simulink model "sf_power_window"  (R2017b)
settings: Solver=FixedStepDiscrete  StartTime=0.0  StopTime=inf  FixedStep=0.1  RelTol=1e-3  EnableMultiTasking=on
PreLoadFcn:
  | %addpath([matlabroot '/toolbox/stateflow/sfdemos']);
  | %addpath([matlabroot '/toolbox/dsp/dsp']);
  | load sf_power_window_buses;
libraries: dspquant2 x1
settings Model: Creator=The MathWorks, Inc.  LastModifiedBy=The MathWorks, Inc.
settings DataIOCC: LimitDataPoints=on  SaveFormat=Array
settings OptimizationCC: LifeSpan=inf
settings DebuggingCC: SolverPrmCheckMsg=warning  AllowSymbolicDim=off  SFUnexpectedBacktrackingDiag=warning  SFNoUnconditionalDefaultTransitionDiag=warning  SFExecutionAtInitializationDiag=none
settings HardwareCC: ProdBitPerPointer=32  ProdBitPerSizeT=32  ProdBitPerPtrDiffT=32  ProdLargestAtomicFloat=None  ProdIntDivRoundTo=Undefined  ProdEndianess=Unspecified  ProdWordSize=32  ProdHWDeviceType=32-bit Generic
settings ModelReferenceCC: PropagateSignalLabelsOutOfModel=off
settings CodeAppCC: StateflowObjectComments=on
settings GRTTargetCC: TargetLangStandard=C89/C90 (ANSI)  GeneratePreprocessorConditionals=Disable all
settings ConfigComp: CovMetricSettings=dw  CovHtmlReporting=on  CovSaveCumulativeToWorkspaceVar=on  CovSaveSingleToWorkspaceVar=on  CovExternalEMLEnable=off  CovSFcnEnable=off

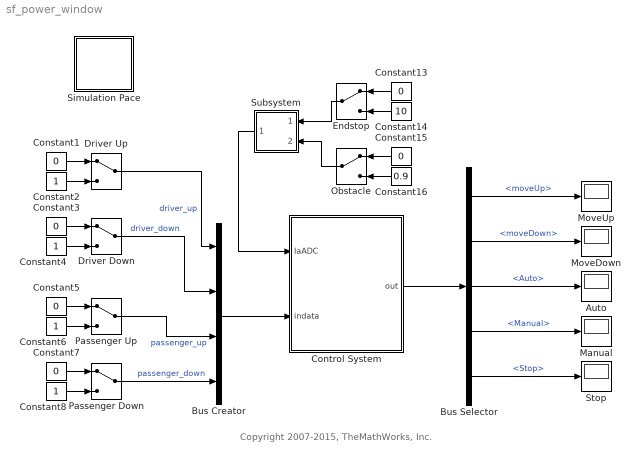
== system sf_power_window ==
  note: Copyright 2007-2015, TheMathWorks, Inc.
  Auto : Display
  Bus Creator : BusCreator  Inputs=4  OutDataTypeStr=Bus: in_busobj  NonVirtualBus=on
  Bus Selector : BusSelector  DialogController=Simulink.DDGSource_BusSelector  OutputSignals=moveUp,moveDown,Auto,Manual,Stop
  Constant{1,3,5,7} (4 alike) : Constant  Value=0  OutDataTypeStr=boolean
  Constant13 : Constant  Value=0
  Constant14 : Constant  Value=10
  Constant15 : Constant  Value=0
  Constant16 : Constant  Value=0.9
  Constant{2,4,6,8} (4 alike) : Constant  OutDataTypeStr=boolean
  Control System : Stateflow chart  TreatAsAtomicUnit=on
  Driver Down : ManualSwitch
  Driver Up : ManualSwitch
  Endstop : ManualSwitch
  Manual : Display
  MoveDown : Display
  MoveUp : Display
  Obstacle : ManualSwitch
  Passenger Down : ManualSwitch
  Passenger Up : ManualSwitch
  Simulation Pace : MATLAB Function  TreatAsAtomicUnit=on
  Stop : Display
  Subsystem : Subsystem
  wires:
  Constant13/1 -> Endstop/1
  Constant14/1 -> Endstop/2
  Constant15/1 -> Obstacle/1
  Constant16/1 -> Obstacle/2
  Endstop/1 -> Subsystem/1(In1)
  Obstacle/1 -> Subsystem/2(In2)
  Constant1/1 -> Driver Up/1
  Constant2/1 -> Driver Up/2
  Constant3/1 -> Driver Down/1
  Constant4/1 -> Driver Down/2
  Constant5/1 -> Passenger Up/1
  Constant6/1 -> Passenger Up/2
  Constant7/1 -> Passenger Down/1
  Constant8/1 -> Passenger Down/2
  Driver Up/1 -> Bus Creator/1  "driver_up"
  Driver Down/1 -> Bus Creator/2  "driver_down"
  Passenger Up/1 -> Bus Creator/3  "passenger_up"
  Passenger Down/1 -> Bus Creator/4  "passenger_down"
  Bus Creator/1 -> Control System/2(indata)
  Subsystem/1(Out1) -> Control System/1(IaADC)
  Control System/1(out) -> Bus Selector/1
  Bus Selector/1 -> MoveUp/1  "<moveUp>"
  Bus Selector/2 -> MoveDown/1  "<moveDown>"
  Bus Selector/3 -> Auto/1  "<Auto>"
  Bus Selector/4 -> Manual/1  "<Manual>"
  Bus Selector/5 -> Stop/1  "<Stop>"

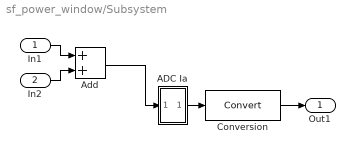
== system sf_power_window/Subsystem ==
  In1 : Inport
  In2 : Inport  Port=2
  ADC Ia : Subsystem  mask(AD Converter){Ts=0.01, peak=3.5, Td=0.005, bits=8}
      mask prompts: Ts "sample time (-1 for inherited)"; Td "delay (-1 for inherited)"
      mask help: Analog (A) to digital (D) converter with sample rate, conversion delay, range, and number of bits used for conversion.
      mask Display:
      | plot([0.5 1.5 1.5 2.5 2.5 3.5 3.5 4.5], [0 0 1 1 2 2 3 3])
      | plot([0 3], [0 3])
  Add : Sum
  Conversion : DataTypeConversion  ConvertRealWorld=Stored Integer (SI)  RndMeth=Nearest  SaturateOnIntegerOverflow=on
  Out1 : Outport
  wires:
  Add/1 -> ADC Ia/1(A)
  ADC Ia/1(D) -> Conversion/1
  In1/1 -> Add/1
  In2/1 -> Add/2
  Conversion/1 -> Out1/1

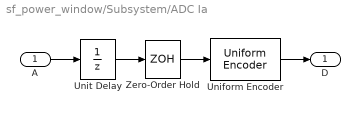
== system sf_power_window/Subsystem/ADC Ia ==
  A : Inport
  Uniform Encoder : dspquant2/Uniform Encoder  peak=peak  bits=bits  otype=Signed integer
      settings: SourceProductName=DSP System Toolbox
  Unit Delay : UnitDelay  SampleTime=0.1
  Zero-Order Hold : ZeroOrderHold  SampleTime=0.1
  D : Outport
  wires:
  A/1 -> Unit Delay/1
  Unit Delay/1 -> Zero-Order Hold/1
  Zero-Order Hold/1 -> Uniform Encoder/1
  Uniform Encoder/1 -> D/1

== matlab function sf_power_window/Simulation Pace ==
function fcn()
pause(0.1);

== stateflow chart sf_power_window/Control System ==
  state Switch [parallel]
    du: switches();
    settings: executionOrder=1
  state Logic [parallel]
    settings: executionOrder=2
    note: Remain in Stop state until a NEUTRAL event triggers Stop.Mode to be Ready.
        | Fail safe time out after continuous movement of more than five seconds.
    state Stop
      en:go.neutral();
      en:out.Stop=true;
      ex:out.Stop=false;
      state Mode [parallel]
        settings: executionOrder=1
        state Waiting
        state Ready
        (default) -> Waiting
        Waiting -> Ready : NEUTRAL
      state Position [parallel]
        settings: executionOrder=2
        state NotSureWhere
        state NearTop
        state NearBottom
        (default) -> NotSureWhere
        (junction 38) -> NearTop [order 1] : [in(EndStop.AtTop)]
        (junction 38) -> NearBottom [order 2]
    state go [group]
      state up [function]
        (default) -> (junction 123) : {out.moveDown = false;
            |  out.moveUp = true;}
      state neutral [function]
        (default) -> (junction 129) : {out.moveUp = false;
            |  out.moveDown = false;}
      state down [function]
        (default) -> (junction 126) : {out.moveUp = false;
            |  out.moveDown = true;}
    state EmergencyDown
      en: go.down();
    state Move
      en: obstacles.init();
      du: obstacles.detect();
      state obstacles [group]
        state detect [function]
          (default) -> (junction 134) : { newIa = cast(Ia*fi(0.96875,1,16,8) + IaADC*fi(0.03125,1,16,8), 'like', newIa);
              |   dIa = newIa-Ia;
              |   Ia = newIa;}
          (junction 134) -> (junction 135) [order 1] : [out.moveUp && Ia > 0.9]
          (junction 135) -> (junction 140) [order 1] : [(dIa >= 0.1)]  % top endstop
          (junction 134) -> (junction 139) [order 2]
          (junction 135) -> (junction 149) [order 2] : {send(OBSTACLE,Move);}
          (junction 140) -> (junction 148) : {send(ENDSTOP,Move);}
          (junction 139) -> (junction 141) [order 1] : [out.moveDown && (Ia < -2.0) && (dIa <= -0.1)]  % bottom endstop
          (junction 139) -> (junction 155) [order 2]
          (junction 141) -> (junction 143) : {send(ENDSTOP,Move);}
        state init [function]
          (default) -> (junction 146) : {Ia=fi(0,1,16,8);}
      state Direction [parallel]
        settings: executionOrder=1
        state Down
          en: go.down();
        state Error
        state Up
          en: go.up();
        Direction -> (junction 28)
        (default) -> Error
        (junction 28) -> Down [order 1] : DOWN
            | [~in(Down)]
        (junction 28) -> (junction 26) [order 2]
        (junction 26) -> Up : UP
            | [~in(Up)]
      state Mode [parallel]
        settings: executionOrder=2
        state Auto
          en:out.Auto=true;
          ex:out.Auto=false;
        state NotSureYet
        state Manual
          en: out.Manual = true;
          ex: out.Manual = false;
        Logic.Move.Mode -> NotSureYet : [in(Direction.Up) || ...
            | in(Direction.Down)]
        (default) -> NotSureYet
        NotSureYet -> Auto [order 2] : NEUTRAL
            | [after(200,msec)]
        NotSureYet -> Manual [order 3] : after(1,sec)
    state EndStop
      state AtTop
        en: go.down();
      state AtBottom
        en: go.up();
      (junction 45) -> AtTop [order 2]
      (junction 45) -> AtBottom [order 1] : [in(Move.Direction.Down)]
    (default) -> Stop
    EmergencyDown -> Stop : [after(1,sec)]
    Move -> EmergencyDown [order 4] : OBSTACLE
    Move -> Stop [order 2] : after(FAILSAFE_TIMEOUT,msec)
    NotSureWhere -> (junction 46) : UP || DOWN
    (junction 46) -> (junction 99)
    NearTop -> (junction 99) : DOWN
    (junction 99) -> (junction 16)
    NearBottom -> (junction 16) : UP
    (junction 16) -> Move : [in(Stop.Mode.Ready)]
    EndStop -> (junction 38) : after(100,msec)
    (junction 95) -> Stop
    Move -> (junction 95) [order 1] : NEUTRAL
        | [in(Move.Mode.Manual)]
    NotSureYet -> (junction 95) [order 1] : NEUTRAL
    Move -> (junction 45) [order 3] : ENDSTOP
  data: dIa temporary fixdt(1,17,8) size=1; newIa temporary fixdt(1,16,8) size=1; Ia local; out output Bus: out_busobj =0; FAILSAFE_TIMEOUT constant uint16 size=1 =4999; IaADC input fixdt(1,8,3) size=1; indata input Bus: in_busobj size=1
  events: OBSTACLE local FUNCTION_CALL_EVENT; NEUTRAL local FUNCTION_CALL_EVENT; ENDSTOP local FUNCTION_CALL_EVENT; UP local FUNCTION_CALL_EVENT; DOWN local FUNCTION_CALL_EVENT
  function switches:
    | function switches
    | 
    | aVarTruthTableCondition_1 = false;
    | aVarTruthTableCondition_2 = false;
    | aVarTruthTableCondition_3 = false;
    | aVarTruthTableCondition_4 = false;
    | 
    | 
    | 
    | aVarTruthTableCondition_1 = logical(indata.driver_up);
    | 
    | 
    | aVarTruthTableCondition_2 = logical(indata.driver_down);
    | 
    | 
    | aVarTruthTableCondition_3 = logical(indata.passenger_up);
    | 
    | 
    | aVarTruthTableCondition_4 = logical(indata.passenger_down);
    | 
    | if (aVarTruthTableCondition_1 && ~aVarTruthTableCondition_2)
    |     aFcnTruthTableAction_1();
    | elseif (~aVarTruthTableCondition_1 && aVarTruthTableCondition_2)
    |     aFcnTruthTableAction_2();
    | elseif (~aVarTruthTableCondition_1 && ~aVarTruthTableCondition_2 && aVarTruthTableCondition_3 && ~aVarTruthTableCondition_4)
    |     aFcnTruthTableAction_1();
    | elseif (~aVarTruthTableCondition_1 && ~aVarTruthTableCondition_2 && ~aVarTruthTableCondition_3 && aVarTruthTableCondition_4)
    |     aFcnTruthTableAction_2();
    | else % Default
    |     aFcnTruthTableAction_3();
    | end
    | 
    | function aFcnTruthTableAction_1()
    | 
    | % Move Up
    | 
    | send(UP,Logic);
    | 
    | function aFcnTruthTableAction_2()
    | 
    | % Move Down
    | 
    | send(DOWN,Logic);
    | 
    | function aFcnTruthTableAction_3()
    | 
    | % Stay Neutral
    | 
    | send(NEUTRAL,Logic);
